simulink model "sampleModel1469"  (R2023a)
settings: Solver=VariableStepAuto  StartTime=0.0  StopTime=10.0  RelTol=1e-3
libraries: hdlsllib x5, simulink x1
settings Model: Creator=user1  LastModifiedBy=user1

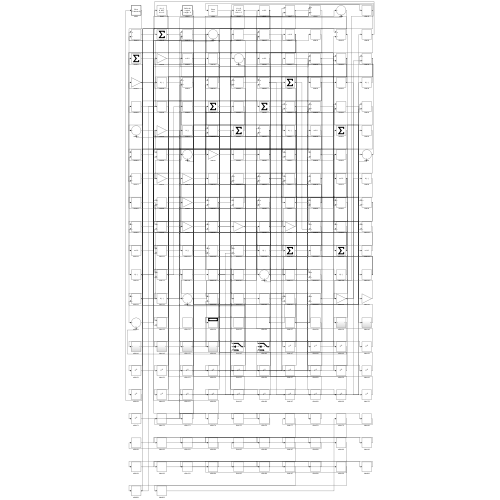
[thumbnail: Simulink's stored preview of the top-level diagram]
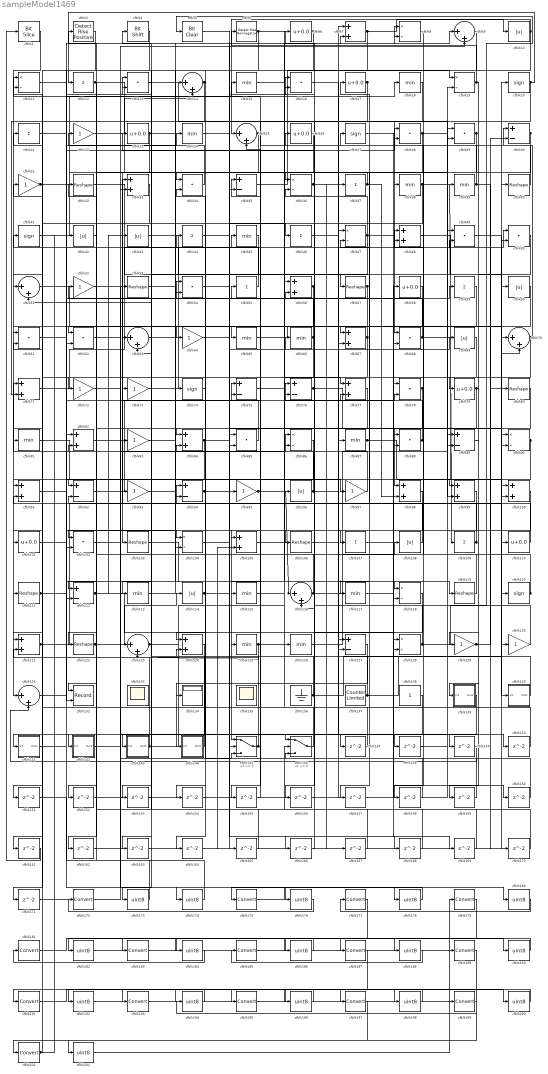
== system sampleModel1469 ==
  cfblk1 : hdlsllib/Logic and Bit Operations/Bit Slice  lidx=7  ridx=0
  cfblk{10,42..43,60,69,96,108,114} (8 alike) : Abs  SaturateOnIntegerOverflow=off
  cfblk{7,33,48,56,67,71,77,82,84,91,98..100,105,121,124} (16 alike) : Sum
  cfblk{6,17,23,26,58,79,101,110} (8 alike) : Bias  Bias=0.0  SaturateOnIntegerOverflow=off
  cfblk{13,16,28..29,34,49..50,54,61..62,68,78,85,88,102} (15 alike) : DotProduct  OutDataTypeStr=Inherit: Inherit via internal rule
  cfblk{32,40,53,57,80,103,106,111,119,122} (10 alike) : Reshape
  cfblk{8,11,19,36,47,86,90,104,118,128} (10 alike) : Product  Inputs=*/  RndMeth=Zero  SaturateOnIntegerOverflow=on
  cfblk{12,21,37,44,46,55,59,107,109} (9 alike) : Sum  Inputs=+
  cfblk{30,35,75..76,89,92,94,112,127} (9 alike) : Sum  Inputs=+-
  cfblk{15,18,24,38..39,45,65..66,81,87,113,115,117,125..126} (15 alike) : MinMax
  cfblk{9,14,25,51,63,70,116,123,131} (9 alike) : Sum  Inputs=|++
  cfblk{20,27,41,74,120} (5 alike) : Signum
  cfblk{22,31,52,64,72..73,83,93,95,97,129..130} (12 alike) : Gain
  cfblk132 : Record  FileSettingsInternal="{\"entries\":[{\"content\":{\"excelSettings\":{\"content\":{},\"type\":\"Streamout.ExcelSettings\"}},\"type\":\"Streamout.FileSettingStorage\",\"uuid\":\"\"}],\"packageUris\":[\"http:\\/\\/schema.mathworks.com\\/mf0\\/streamout_blocks\\/R2020a\"],\"version\":\"1.0\"}"  Layout=[1 1]  SignalsInternal="{\"entries\":[{\"content\":{\"signals\":[{\"content\":{\"blockPath\":[],\"dimensions\":[1],\"domain\":\"\",\"lineColor\":\"#a2142f\",\"plots\":[1],\"port\":1,\"signalID\":954,\"signalName\":\"XY Graph:1\"},\"type\":\"RecordBlkView.Signal\",\"uuid\":\"\"},{\"content\":{\"blockPath\":[],\"dimensions\":[1],\"domain\":\"\",\"lineColor\":\"#139fff\",\"plots\":[1],\"port\":2,\"signalID\":957,\"signalName\":\"XY Graph:2\"},\"type\":\"RecordBlkView.Signal\",\"uuid\":\"\"}]},\"type\":\"RecordBlkView.InputSignals\",\"uuid\":\"\"}],\"packageUris\":[\"http:\\/\\/schema.mathworks.com\\/mf0\\/streamout_blocks\\/R2020a\"],\"version\":\"1.0\"}"  VisualizationBindings="{\"xyplotplugin\":{\"info\":[{\"series\":[{\"bindingParametersList\":[{\"parameter\":\"X-Axis\",\"signalID\":954,\"signalName\":\"XY Graph:1\"},{\"parameter\":\"Y-Axis\",\"signalID\":957,\"signalName\":\"XY Graph:2\"}],\"seriesID\":62886}],\"subplotID\":1}]}}"  CompatibilityTag=XY  st=-1
  cfblk133 : Scope
      settings: Floating=on
  cfblk134 : Display
  cfblk135 : Scope
      settings: Floating=on
  cfblk136 : Ground
  cfblk137 : hdlsllib/Sources/Counter Limited  uplimit=7  tsamp=-1
  cfblk138 : Constant  SampleTime=-1
  cfblk139 : Subsystem
      settings: LibrarySourceBlock=|
      | hdlsllib/Ports &
      | Subsystems/Subsystem
  cfblk140 : Subsystem
      settings: LibrarySourceBlock=|
      | hdlsllib/Ports &
      | Subsystems/Subsystem
  cfblk141 : Subsystem
      settings: LibrarySourceBlock=|
      | hdlsllib/Ports &
      | Subsystems/Subsystem
  cfblk142 : Subsystem
      settings: LibrarySourceBlock=|
      | hdlsllib/Ports &
      | Subsystems/Subsystem
  cfblk143 : Subsystem
      settings: LibrarySourceBlock=|
      | hdlsllib/Ports &
      | Subsystems/Subsystem
  cfblk144 : Subsystem
      settings: LibrarySourceBlock=|
      | hdlsllib/Ports &
      | Subsystems/Subsystem
  cfblk145 : Switch  SaturateOnIntegerOverflow=off  InputSameDT=off
  cfblk146 : Switch  SaturateOnIntegerOverflow=off  InputSameDT=off
  cfblk{147..171} (25 alike) : Delay  SampleTime=1
  cfblk{172,175,177,179,181,183,185,187,189,191,193,195,197,199,201} (15 alike) : DataTypeConversion  SaturateOnIntegerOverflow=off  RndMeth=Floor
  cfblk{173..174,176,178,180,182,184,186,188,190,192,194,196,198,200,202} (16 alike) : DataTypeConversion  OutDataTypeStr=uint8  SaturateOnIntegerOverflow=off  RndMeth=Floor
  cfblk2 : hdlsllib/Logic and Bit Operations/Detect Rise Positive  vinit=0  OutDataTypeStr=boolean
  cfblk3 : hdlsllib/Logic and Bit Operations/Bit Shift  mode=Shift Left Logical  N=0
  cfblk4 : simulink/Logic and Bit Operations/Bit Clear  iBit=0
      settings: LibrarySourceBlock=|
      | hdlsllib/Logic and Bit
      | Operations/Bit Clear
  cfblk5 : hdlsllib/Logic and Bit Operations/Detect Rise Nonnegative  vinit=0  OutDataTypeStr=boolean
  wires:
  cfblk18/1 -> cfblk68/1
  cfblk35/1 -> cfblk19/1
  cfblk23/1 -> cfblk103/1, cfblk118/2
  cfblk32/1 -> cfblk57/1
  cfblk94/1 -> cfblk95/1, cfblk66/1
  cfblk67/1 -> cfblk62/1, cfblk151/1
  cfblk34/1 -> cfblk131/1
  cfblk73/1 -> cfblk45/1
  cfblk129/1 -> cfblk80/1, cfblk30/2
  cfblk10/1 -> cfblk25/1, cfblk94/2
  cfblk1/1 -> cfblk111/1
  cfblk122/1 -> cfblk114/1, cfblk9/2
  cfblk33/1 -> cfblk92/1
  cfblk146/1 -> cfblk54/1
  cfblk128/1 -> cfblk4/1, cfblk23/1
  cfblk121/1 -> cfblk20/1, cfblk77/2
  cfblk20/1 -> cfblk12/1, cfblk36/1
  cfblk71/1 -> cfblk50/1
  cfblk103/1 -> cfblk145/1
  cfblk80/1 -> cfblk132/1
  cfblk39/1 -> cfblk11/1, cfblk170/1
  cfblk46/1 -> cfblk87/1
  cfblk11/1 -> cfblk119/1
  cfblk56/1 -> cfblk65/1, cfblk102/2
  cfblk38/1 -> cfblk109/1, cfblk62/2, cfblk161/1
  cfblk79/1 -> cfblk157/1, cfblk158/1, cfblk159/1
  cfblk55/1 -> cfblk41/1
  cfblk14/1 -> cfblk153/1, cfblk154/1
  cfblk87/1 -> cfblk17/1, cfblk100/2
  cfblk107/1 -> cfblk58/1
  cfblk114/1 -> cfblk105/2, cfblk165/1, cfblk166/1
  cfblk106/1 -> cfblk37/1
  cfblk60/1 -> cfblk112/1
  cfblk84/1 -> cfblk91/1, cfblk8/2
  cfblk9/1 -> cfblk84/1
  cfblk29/1 -> cfblk88/2, cfblk147/1
  cfblk61/1 -> cfblk55/1
  cfblk92/1 -> cfblk76/1
  cfblk43/1 -> cfblk90/1
  cfblk145/1 -> cfblk44/1, cfblk121/2
  cfblk100/1 -> cfblk125/1
  cfblk41/1 -> cfblk15/1
  cfblk91/1 -> cfblk59/1
  cfblk102/1 -> cfblk86/1
  cfblk144/1(Out1) -> cfblk3/1
  cfblk57/1 -> cfblk64/1, cfblk81/1
  cfblk130/1 -> cfblk94/1
  cfblk138/1 -> cfblk143/1(In1)
  cfblk50/1 -> cfblk99/1
  cfblk74/1 -> cfblk54/2
  cfblk83/1 -> cfblk74/1
  cfblk66/1 -> cfblk86/2, cfblk32/1
  cfblk137/1 -> cfblk50/2, cfblk60/1, cfblk51/2
  cfblk25/1 -> cfblk142/1(In1), cfblk113/1
  cfblk95/1 -> cfblk116/1, cfblk75/2
  cfblk26/1 -> cfblk102/1
  cfblk141/1(Out1) -> cfblk9/1
  cfblk125/1 -> cfblk126/1, cfblk123/2
  cfblk76/1 -> cfblk110/1, cfblk48/2
  cfblk19/1 -> cfblk5/1, cfblk79/1
  cfblk124/1 -> cfblk141/1(In1)
  cfblk68/1 -> cfblk120/1, cfblk35/1
  cfblk7/1 -> cfblk10/1, cfblk51/1
  cfblk123/1 -> cfblk69/1, cfblk163/1
  cfblk85/1 -> cfblk33/1
  cfblk111/1 -> cfblk24/1, cfblk28/2
  cfblk142/1(Out1) -> cfblk145/3
  cfblk86/1 -> cfblk105/1
  cfblk89/1 -> cfblk139/1(In1)
  cfblk31/1 -> cfblk38/1, cfblk97/1
  cfblk101/1 -> cfblk18/1
  cfblk78/1 -> cfblk98/1, cfblk48/1
  cfblk115/1 -> cfblk8/1
  cfblk44/1 -> cfblk46/1
  cfblk4/1 -> cfblk90/2
  cfblk120/1 -> cfblk16/1, cfblk93/1, cfblk28/1
  cfblk51/1 -> cfblk130/1
  cfblk143/1(Out1) -> cfblk96/1, cfblk91/2
  cfblk30/1 -> cfblk146/1, cfblk67/2
  cfblk24/1 -> cfblk85/1
  cfblk112/1 -> cfblk128/2, cfblk43/1
  cfblk69/1 -> cfblk116/2
  cfblk131/1 -> cfblk13/1
  cfblk110/1 -> cfblk73/1
  cfblk5/1 -> cfblk132/2, cfblk118/1
  cfblk13/1 -> cfblk39/1
  cfblk40/1 -> cfblk26/1
  cfblk42/1 -> cfblk72/1
  cfblk90/1 -> cfblk106/1, cfblk104/2
  cfblk88/1 -> cfblk6/1, cfblk47/2
  cfblk3/1 -> cfblk112/2
  cfblk126/1 -> cfblk108/1
  cfblk81/1 -> cfblk123/1
  cfblk49/1 -> cfblk70/1
  cfblk28/1 -> cfblk99/2, cfblk35/2
  cfblk59/1 -> cfblk101/1
  cfblk12/1 -> cfblk89/1, cfblk122/1
  cfblk17/1 -> cfblk115/1, cfblk124/1, cfblk71/2
  cfblk136/1 -> cfblk40/1, cfblk134/1, cfblk124/2
  cfblk75/1 -> cfblk77/1
  cfblk108/1 -> cfblk31/1
  cfblk104/1 -> cfblk16/2
  cfblk2/1 -> cfblk61/1
  cfblk96/1 -> cfblk47/1, cfblk52/1
  cfblk70/1 -> cfblk129/1, cfblk30/1
  cfblk109/1 -> cfblk27/1, cfblk21/1
  cfblk93/1 -> cfblk56/2
  cfblk15/1 -> cfblk29/2
  cfblk105/1 -> cfblk78/2
  cfblk119/1 -> cfblk2/1
  cfblk6/1 -> cfblk63/1, cfblk121/1
  cfblk140/1(Out1) -> cfblk22/1
  cfblk113/1 -> cfblk14/1
  cfblk65/1 -> cfblk67/1
  cfblk52/1 -> cfblk83/1
  cfblk116/1 -> cfblk19/2, cfblk75/1
  cfblk22/1 -> cfblk14/2
  cfblk36/1 -> cfblk89/2, cfblk167/1
  cfblk127/1 -> cfblk144/1(In1)
  cfblk37/1 -> cfblk34/1, cfblk98/2, cfblk107/1
  cfblk48/1 -> cfblk140/1(In1)
  cfblk21/1 -> cfblk104/1
  cfblk53/1 -> cfblk49/2
  cfblk117/1 -> cfblk68/2
  cfblk54/1 -> cfblk127/2
  cfblk97/1 -> cfblk71/1
  cfblk72/1 -> cfblk53/1
  cfblk47/1 -> cfblk63/2, cfblk117/1, cfblk36/2, cfblk169/1
  cfblk63/1 -> cfblk7/2
  cfblk147/1 -> cfblk11/2
  cfblk8/1 -> cfblk148/1
  cfblk148/1 -> cfblk49/1
  cfblk16/1 -> cfblk149/1
  cfblk149/1 -> cfblk131/2
  cfblk62/1 -> cfblk150/1
  cfblk150/1 -> cfblk56/1
  cfblk98/1 -> cfblk152/1
  cfblk152/1 -> cfblk127/1
  cfblk153/1 -> cfblk78/1
  cfblk154/1 -> cfblk88/1
  cfblk99/1 -> cfblk155/1
  cfblk155/1 -> cfblk25/2
  cfblk118/1 -> cfblk156/1
  cfblk156/1 -> cfblk7/1
  cfblk157/1 -> cfblk29/1
  cfblk158/1 -> cfblk34/2
  cfblk159/1 -> cfblk84/2
  cfblk27/1 -> cfblk160/1
  cfblk160/1 -> cfblk128/1
  cfblk161/1 -> cfblk1/1
  cfblk77/1 -> cfblk162/1
  cfblk162/1 -> cfblk100/1
  cfblk163/1 -> cfblk85/2
  cfblk139/1(Out1) -> cfblk164/1
  cfblk164/1 -> cfblk70/2
  cfblk165/1 -> cfblk145/2
  cfblk166/1 -> cfblk76/2
  cfblk167/1 -> cfblk146/3
  cfblk64/1 -> cfblk168/1
  cfblk168/1 -> cfblk146/2
  cfblk169/1 -> cfblk92/2
  cfblk170/1 -> cfblk13/2
  cfblk58/1 -> cfblk171/1
  cfblk171/1 -> cfblk33/2
  cfblk45/1 -> cfblk173/1
  cfblk173/1 -> cfblk82/1
  cfblk151/1 -> cfblk174/1
  cfblk174/1 -> cfblk82/2
  cfblk82/1 -> cfblk176/1
  cfblk176/1 -> cfblk172/1
  cfblk172/1 -> cfblk178/1
  cfblk178/1 -> cfblk175/1
  cfblk175/1 -> cfblk180/1
  cfblk180/1 -> cfblk177/1
  cfblk177/1 -> cfblk182/1
  cfblk182/1 -> cfblk179/1
  cfblk179/1 -> cfblk184/1
  cfblk184/1 -> cfblk181/1
  cfblk181/1 -> cfblk186/1
  cfblk186/1 -> cfblk183/1
  cfblk183/1 -> cfblk188/1
  cfblk188/1 -> cfblk185/1
  cfblk185/1 -> cfblk190/1
  cfblk190/1 -> cfblk187/1
  cfblk187/1 -> cfblk192/1
  cfblk192/1 -> cfblk189/1
  cfblk189/1 -> cfblk194/1
  cfblk194/1 -> cfblk191/1
  cfblk191/1 -> cfblk196/1
  cfblk196/1 -> cfblk193/1
  cfblk193/1 -> cfblk198/1
  cfblk198/1 -> cfblk195/1
  cfblk199/1 -> cfblk201/1
  cfblk195/1 -> cfblk200/1
  cfblk200/1 -> cfblk197/1
  cfblk201/1 -> cfblk61/2, cfblk42/1
  cfblk197/1 -> cfblk202/1
  cfblk202/1 -> cfblk199/1

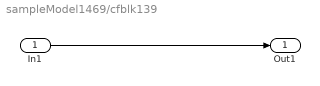
== system sampleModel1469/cfblk139 ==
  In1 : Inport
  Out1 : Outport
  wires:
  In1/1 -> Out1/1

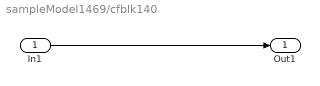
== system sampleModel1469/cfblk140 ==
  In1 : Inport
  Out1 : Outport
  wires:
  In1/1 -> Out1/1

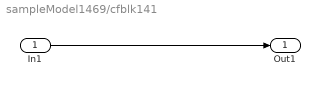
== system sampleModel1469/cfblk141 ==
  In1 : Inport
  Out1 : Outport
  wires:
  In1/1 -> Out1/1

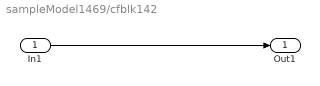
== system sampleModel1469/cfblk142 ==
  In1 : Inport
  Out1 : Outport
  wires:
  In1/1 -> Out1/1

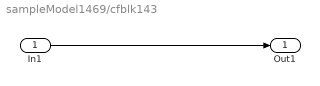
== system sampleModel1469/cfblk143 ==
  In1 : Inport
  Out1 : Outport
  wires:
  In1/1 -> Out1/1

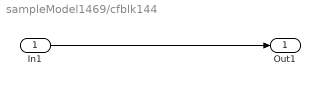
== system sampleModel1469/cfblk144 ==
  In1 : Inport
  Out1 : Outport
  wires:
  In1/1 -> Out1/1
